simulink subsystem "pitch_parameters_bus"  (R2022b)
settings: Solver=VariableStepAuto  StartTime=0.0  StopTime=10.0  RelTol=1e-3
settings Model: Creator=User  LastModifiedBy=User

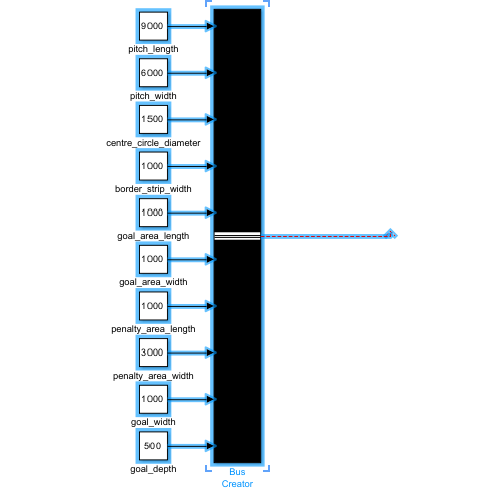
[thumbnail: Simulink's stored preview of the top-level diagram]
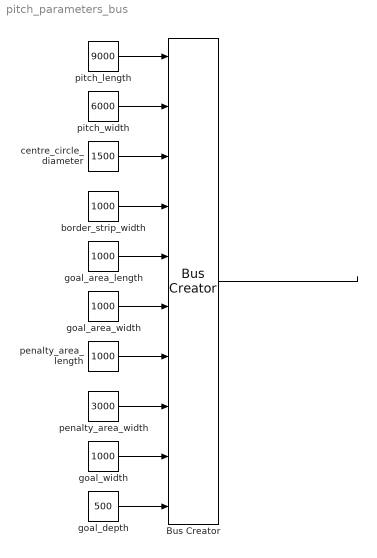
== system pitch_parameters_bus ==
  Bus Creator : BusCreator  Inputs=10
  border_strip_width : Constant  Value=1000
  centre_circle_diameter : Constant  Value=1500
  goal_area_length : Constant  Value=1000
  goal_area_width : Constant  Value=1000
  goal_depth : Constant  Value=500
  goal_width : Constant  Value=1000
  penalty_area_length : Constant  Value=1000
  penalty_area_width : Constant  Value=3000
  pitch_length : Constant  Value=9000
  pitch_width : Constant  Value=6000
  wires:
  goal_depth/1 -> Bus Creator/10
  goal_width/1 -> Bus Creator/9
  penalty_area_width/1 -> Bus Creator/8
  penalty_area_length/1 -> Bus Creator/7
  goal_area_width/1 -> Bus Creator/6
  goal_area_length/1 -> Bus Creator/5
  border_strip_width/1 -> Bus Creator/4
  centre_circle_diameter/1 -> Bus Creator/3
  pitch_width/1 -> Bus Creator/2
  pitch_length/1 -> Bus Creator/1
  Bus Creator/1 -> ?
